simulink model "lab3_linear_2023a"  (R2023a)
settings: Solver=VariableStepAuto  StartTime=0.0  StopTime=10.0  RelTol=1e-10  AbsTol=1e-10
values from neighbouring files (symbols this model uses):
  A = double(A)    [lab3.m]
  B = double(B)    [lab3.m]
  K = -K_lqr2    [lab3.m]
  x0 = [0; 0; n*pi/24; 0]    [lab3.m]
settings Model: Creator=dell  LastModifiedBy=dell

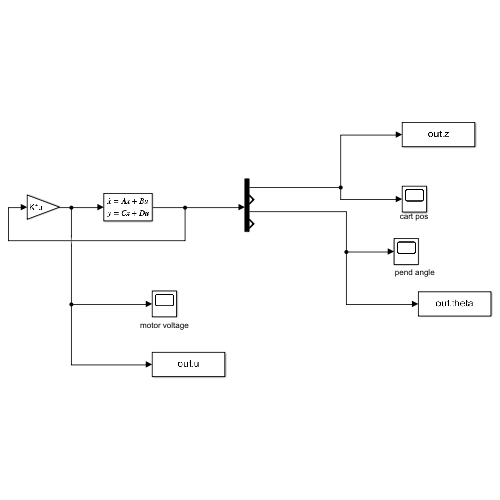
[thumbnail: Simulink's stored preview of the top-level diagram]
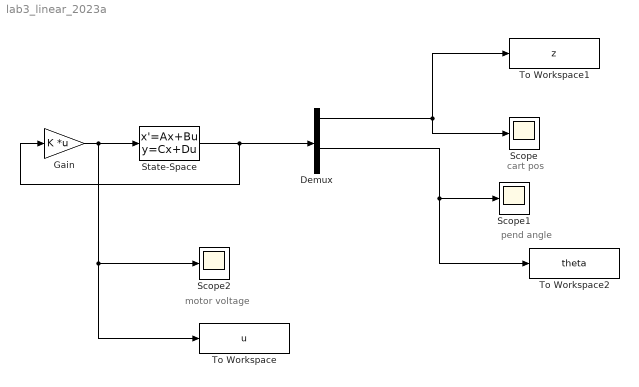
== system lab3_linear_2023a ==
  note: motor voltage
  note: pend angle
  note: cart pos
  Demux : Demux
  Gain : Gain  Gain=K  Multiplication=Matrix(K*u)
  Scope : Scope
  Scope1 : Scope
  Scope2 : Scope
  State-Space : StateSpace  A=A  B=B  C=eye(4)  D=zeros(4, 1)  InitialCondition=x0
  To Workspace : ToWorkspace  VariableName=u  SaveFormat=Timeseries  SampleTime=-1
  To Workspace1 : ToWorkspace  VariableName=z  SaveFormat=Timeseries  SampleTime=-1
  To Workspace2 : ToWorkspace  VariableName=theta  SaveFormat=Timeseries  SampleTime=-1
  wires:
  Gain/1 -> To Workspace/1, Scope2/1, State-Space/1
  State-Space/1 -> Gain/1, Demux/1
  Demux/1 -> To Workspace1/1, Scope/1
  Demux/3 -> To Workspace2/1, Scope1/1
